simulink model "htt_ngang"  (Simulink 8.3)
settings: Solver=ode45  StartTime=0.0  StopTime=10  FixedStep=0.05  RelTol=1e-3
values from neighbouring files (symbols this model uses):
  Af = [msf 0 0 0 ... (first row only)    [main2.m]
  Bf = [2*Ksf 0 -2*Ksf 0 ... (first row only)    [main2.m]
  Cf = [2*Csf 0 -2*Csf 0 ... (first row only)    [main2.m]
  Ctf = 293250    [main2.m]
  duf = 1.5/2    (= 0.75)    [main2.m]
  Ktf = 26960    [main2.m]
settings Model: Creator=HIENANH  LastModifiedBy=HIENANH
settings DebuggingCC: FcnCallInpInsideContextMsg=EnableAllAsWarning  StateNameClashWarn=none

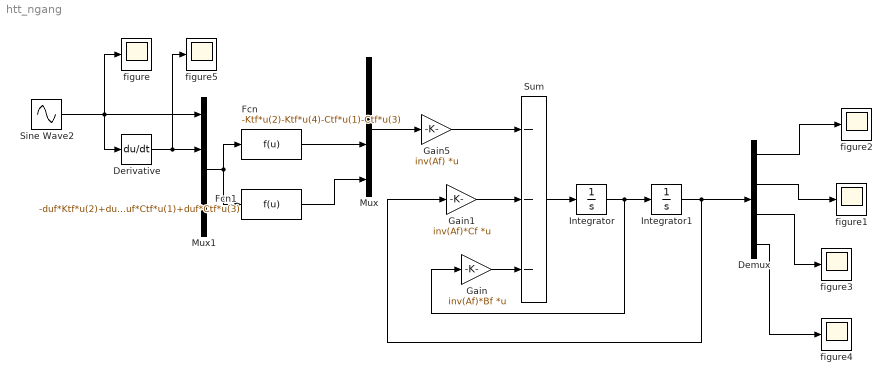
== system htt_ngang ==
  Demux : Demux
  Derivative : Derivative
  Fcn : Fcn  Expr=-Ktf*u(2)-Ktf*u(4)-Ctf*u(1)-Ctf*u(3)
  Fcn1 : Fcn  Expr=-duf*Ktf*u(2)+duf*Ktf*u(4)-duf*Ctf*u(1)+duf*Ctf*u(3)
  Gain : Gain  Gain=inv(Af)*Bf  Multiplication=Matrix(K*u)
  Gain1 : Gain  Gain=inv(Af)*Cf  Multiplication=Matrix(K*u)
  Gain5 : Gain  Gain=inv(Af)  Multiplication=Matrix(K*u)
  Integrator : Integrator
  Integrator1 : Integrator
  Mux : Mux
  Mux1 : Mux
  Sine Wave2 : Sin  Amplitude=0.1  Frequency=10  SampleTime=0
  Sum : Sum  Inputs=---
  figure{,1..5} (6 alike) : Scope
      figure settings: YMin=0  YMax=0.07  SaveName=qLf1
      figure1 settings: YMin=0  YMax=0.07  SaveName=xf1
      figure2 settings: YMin=0  YMax=0.07  SaveName=xf
      figure3 settings: YMin=0  YMax=0.07  SaveName=xf2
      figure4 settings: YMin=0  YMax=0.07  SaveName=xf3
      figure5 settings: YMin=0  YMax=0.07  SaveName=dqLf1
  wires:
  Integrator/1 -> Gain/1, Integrator1/1
  Integrator1/1 -> Demux/1, Gain1/1
  Sine Wave2/1 -> figure/1, Derivative/1, Mux1/1
  Fcn/1 -> Mux/3
  Fcn1/1 -> Mux/4
  Derivative/1 -> figure5/1, Mux1/2
  Mux1/1 -> Fcn1/1, Fcn/1
  Mux/1 -> Gain5/1
  Sum/1 -> Integrator/1
  Gain/1 -> Sum/3
  Gain1/1 -> Sum/2
  Gain5/1 -> Sum/1
  Demux/1 -> figure2/1
  Demux/2 -> figure1/1
  Demux/3 -> figure3/1
  Demux/4 -> figure4/1
